simulink model "helicopter_LQR_21b"  (R2021b)
settings: Solver=ode45  StartTime=0.0  StopTime=60  RelTol=1e-3
InitFcn:
  | hwinit
StopFcn:
  | helicoptertest_plot
values from neighbouring files (symbols this model uses):
  adingain = [pitchgain 1 yawgain 1]    [hwinit.m]
  adinoffs = [pitchoffs 0 yawoffs 0]    [hwinit.m]
  angle_ref = neg.mean.pitch(idx)    [hwinit.m]
  angVel_ref = neg.mean.angular_velocity(idx)    [hwinit.m]
  h = 0.001    [hwinit.m]
  input_ref = -0.5    [hwinit.m]
  K_LQR_neg = lqr(helicopterSysID_neg.A,helicopterSysID_neg.B,Q_LQR_neg,R_LQR_neg,0)    [hwinit.m]
  K_LQR_pos = lqr(helicopterSysID_pos.A,helicopterSysID_pos.B,Q_LQR_pos,R_LQR_pos,0)    [hwinit.m]
  Ki_neg = 1    [hwinit.m]
  Ki_pos = 5    [hwinit.m]
undefined symbols (not defined in the file or in its folder): helicopterSysID_neg, helicopterSysID_pos, HeliMexHandle, L_neg, L_pos
libraries: dspfdesign x1
settings Model: Creator=fkzhang  LastModifiedBy=morhun
settings SolverCC: AlgebraicLoopSolver=TrustRegion
settings DataIOCC: LimitDataPoints=on  SaveFormat=Array  ReturnWorkspaceOutputs=off
settings OptimizationCC: BlockReduction=off  BooleanDataType=off  LifeSpan=inf
settings DebuggingCC: SaveWithParameterizedLinksMsg=none  UnderspecifiedInitializationDetection=Classic  MergeDetectMultiDrivingBlocksExec=none  SignalResolutionControl=TryResolveAllWithWarning  AllowSymbolicDim=off  SFUnexpectedBacktrackingDiag=warning  SFNoUnconditionalDefaultTransitionDiag=warning  SFExecutionAtInitializationDiag=none  ArithmeticOperatorsInVariantConditions=warning
settings HardwareCC: ProdBitPerPointer=32  ProdBitPerSizeT=32  ProdBitPerPtrDiffT=32  ProdLargestAtomicFloat=None  ProdIntDivRoundTo=Undefined  ProdEndianess=Unspecified  ProdWordSize=32  ProdHWDeviceType=32-bit Generic  TargetUnknown=on
settings ModelReferenceCC: PropagateSignalLabelsOutOfModel=off
settings SFSimCC: SimUseLocalCustomCode=off  CustomCodeUndefinedFunction=UseInterfaceOnly
settings RTWCC: RTWUseLocalCustomCode=off
settings CodeAppCC: StateflowObjectComments=on
settings GRTTargetCC: TargetLangStandard=C89/C90 (ANSI)
settings ConfigComp: CovMetricSettings=dw  CovSaveCumulativeToWorkspaceVar=on  CovSaveSingleToWorkspaceVar=on  CovExternalEMLEnable=off  CovSFcnEnable=off

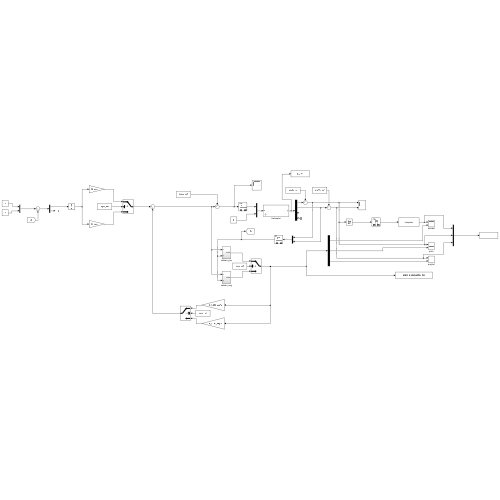
[thumbnail: Simulink's stored preview of the top-level diagram]
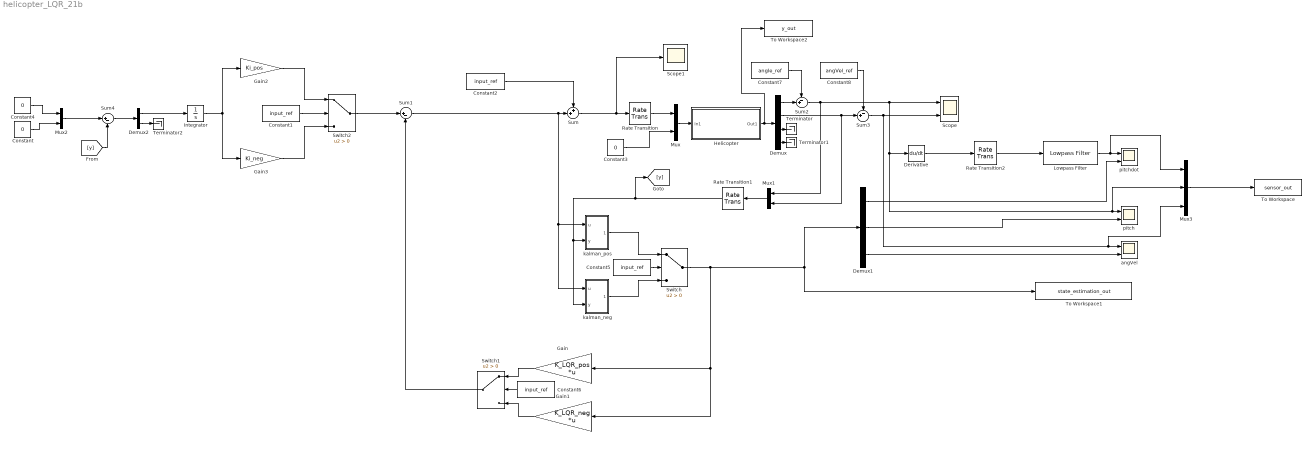
== system helicopter_LQR_21b ==
  Constant : Constant  Value=0
  Constant{1..2,5..6} (4 alike) : Constant  Value=input_ref
  Constant3 : Constant  Value=0
  Constant4 : Constant  Value=0
  Constant7 : Constant  Value=angle_ref
  Constant8 : Constant  Value=angVel_ref
  Demux : Demux
  Demux1 : Demux  Outputs=3
  Demux2 : Demux  Outputs=2
  Derivative : Derivative
  Gain : Gain  Gain=K_LQR_pos  Multiplication=Matrix(K*u)
  Gain1 : Gain  Gain=K_LQR_neg  Multiplication=Matrix(K*u)
  Gain2 : Gain  Gain=Ki_pos
  Gain3 : Gain  Gain=Ki_neg
  Helicopter : Subsystem  mask{Ts=h}
      mask prompts: Ts "sampletime"
      mask init:
      | sf_heli_init
      mask Display:
      | port_label('input',1,'u');
      | port_label('output',1,'y');
  Integrator : Integrator
  Lowpass Filter : dspfdesign/Lowpass Filter  FilterType=FIR  DesignForMinimumOrder=on  FilterOrder=50  PassbandFrequency=1  StopbandFrequency=10  PassbandRipple=0.1  StopbandAttenuation=80  InheritSampleRate=off  SampleRate=1000  SimulateUsing=Interpreted execution  roundingMode=Floor  coeffsDataTypeStr=fixdt(1,16)
  Mux : Mux  Inputs=2
  Mux1 : Mux  Inputs=2
  Mux2 : Mux  Inputs=2
  Mux3 : Mux  Inputs=3
  Rate Transition : RateTransition  OutPortSampleTime=h
  Rate Transition1 : RateTransition
  Rate Transition2 : RateTransition  OutPortSampleTime=h
  Scope : Scope  NumInputPorts=2
  Scope1 : Scope
  Sum : Sum  Inputs=++|
  Sum1 : Sum  Inputs=|+-
  Sum2 : Sum  Inputs=-+|
  Sum3 : Sum  Inputs=-+|
  Sum4 : Sum  Inputs=|+-
  Switch : Switch  Criteria=u2 > Threshold
  Switch1 : Switch  Criteria=u2 > Threshold
  Switch2 : Switch  Criteria=u2 > Threshold
  Terminator : Terminator
  Terminator1 : Terminator
  Terminator2 : Terminator
  To Workspace : ToWorkspace  VariableName=sensor_out  SaveFormat=Timeseries  SampleTime=-1
  To Workspace1 : ToWorkspace  VariableName=state_estimation_out  SaveFormat=Timeseries  SampleTime=-1
  To Workspace2 : ToWorkspace  VariableName=y_out  SaveFormat=Timeseries  SampleTime=-1
  angVel : Scope  NumInputPorts=2
  kalman_neg : Subsystem
  kalman_pos : Subsystem
  pitch : Scope  NumInputPorts=2
  pitchdot : Scope  NumInputPorts=2
  wires:
  Helicopter/1(Out1) -> To Workspace2/1, Demux/1
  Mux/1 -> Helicopter/1(In1)
  Constant3/1 -> Mux/2
  Sum1/1 -> kalman_neg/1(u), kalman_pos/1(u), Sum/2
  Switch/1 -> Gain1/1, Gain/1, Demux1/1, To Workspace1/1
  Demux/3 -> Terminator/1
  Demux/4 -> Terminator1/1
  Demux/1 -> Sum2/2
  Demux/2 -> Mux1/2, Sum3/2
  Constant7/1 -> Sum2/1
  Constant8/1 -> Sum3/1
  kalman_pos/1(xhat) -> Switch/1
  kalman_neg/1(xhat) -> Switch/3
  Rate Transition2/1 -> Lowpass Filter/1
  Derivative/1 -> Rate Transition2/1
  Mux1/1 -> Rate Transition1/1
  Rate Transition1/1 -> [y], kalman_neg/2(y), kalman_pos/2(y)
  Demux1/1 -> pitchdot/2
  Demux1/2 -> pitch/2
  Demux1/3 -> angVel/2
  Rate Transition/1 -> Mux/1
  Gain/1 -> Switch1/1
  Gain1/1 -> Switch1/3
  Switch1/1 -> Sum1/2
  [y] -> Sum4/2
  Sum4/1 -> Demux2/1
  Demux2/2 -> Terminator2/1
  Demux2/1 -> Integrator/1
  Mux2/1 -> Sum4/1
  Constant/1 -> Mux2/2
  Gain2/1 -> Switch2/1
  Gain3/1 -> Switch2/3
  Constant1/1 -> Switch2/2
  Integrator/1 -> Gain2/1, Gain3/1
  Switch2/1 -> Sum1/1
  Lowpass Filter/1 -> Mux3/1, pitchdot/1
  Mux3/1 -> To Workspace/1
  Sum3/1 -> Mux3/3, angVel/1, Scope/2
  Sum2/1 -> Mux1/1, Mux3/2, pitch/1, Derivative/1, Scope/1
  Constant5/1 -> Switch/2
  Constant6/1 -> Switch1/2
  Constant4/1 -> Mux2/1
  Constant2/1 -> Sum/1
  Sum/1 -> Scope1/1, Rate Transition/1

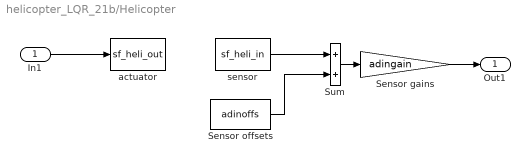
== system helicopter_LQR_21b/Helicopter ==
  In1 : Inport
  Sensor gains : Gain  Gain=adingain
  Sensor offsets : Constant  Value=adinoffs
  Sum : Sum
  actuator : M-S-Function  FunctionName=sf_heli_out  Parameters=HeliMexHandle,Ts
  sensor : M-S-Function  FunctionName=sf_heli_in  Parameters=HeliMexHandle
  Out1 : Outport
  wires:
  sensor/1 -> Sum/1
  In1/1 -> actuator/1
  Sensor offsets/1 -> Sum/2
  Sum/1 -> Sensor gains/1
  Sensor gains/1 -> Out1/1

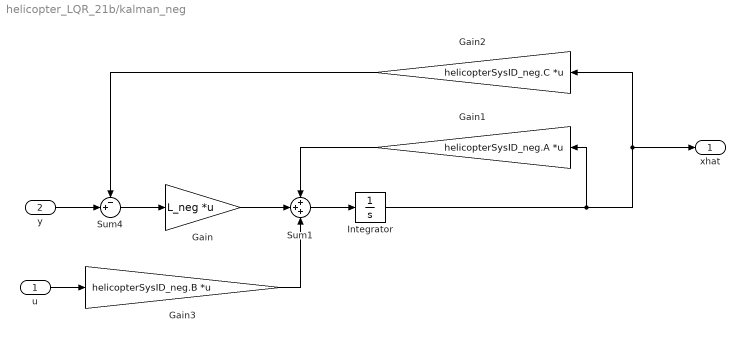
== system helicopter_LQR_21b/kalman_neg ==
  u : Inport
  y : Inport  Port=2
  Gain : Gain  Gain=L_neg  Multiplication=Matrix(K*u)
  Gain1 : Gain  Gain=helicopterSysID_neg.A  Multiplication=Matrix(K*u)
  Gain2 : Gain  Gain=helicopterSysID_neg.C  Multiplication=Matrix(K*u)
  Gain3 : Gain  Gain=helicopterSysID_neg.B  Multiplication=Matrix(K*u)
  Integrator : Integrator  InitialCondition=[0 ; -angle_ref ; -angVel_ref]
  Sum1 : Sum  Inputs=+++
  Sum4 : Sum  Inputs=-+|
  xhat : Outport
  wires:
  Integrator/1 -> Gain1/1, xhat/1, Gain2/1
  y/1 -> Sum4/2
  Sum4/1 -> Gain/1
  u/1 -> Gain3/1
  Gain3/1 -> Sum1/3
  Gain/1 -> Sum1/2
  Sum1/1 -> Integrator/1
  Gain1/1 -> Sum1/1
  Gain2/1 -> Sum4/1

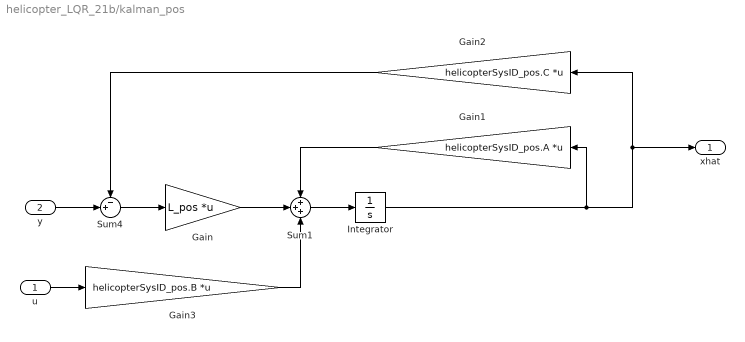
== system helicopter_LQR_21b/kalman_pos ==
  u : Inport
  y : Inport  Port=2
  Gain : Gain  Gain=L_pos  Multiplication=Matrix(K*u)
  Gain1 : Gain  Gain=helicopterSysID_pos.A  Multiplication=Matrix(K*u)
  Gain2 : Gain  Gain=helicopterSysID_pos.C  Multiplication=Matrix(K*u)
  Gain3 : Gain  Gain=helicopterSysID_pos.B  Multiplication=Matrix(K*u)
  Integrator : Integrator  InitialCondition=[0 ; -angle_ref ; -angVel_ref]
  Sum1 : Sum  Inputs=+++
  Sum4 : Sum  Inputs=-+|
  xhat : Outport
  wires:
  Integrator/1 -> Gain1/1, xhat/1, Gain2/1
  y/1 -> Sum4/2
  Sum4/1 -> Gain/1
  u/1 -> Gain3/1
  Gain3/1 -> Sum1/3
  Gain/1 -> Sum1/2
  Sum1/1 -> Integrator/1
  Gain1/1 -> Sum1/1
  Gain2/1 -> Sum4/1
